simulink model "Systeem_Identificatie_Hardware_Code"  (R2018b)
settings: Solver=FixedStepDiscrete  StartTime=0.0  StopTime=1000  FixedStep=1/100000  RelTol=1e-3  EnableMultiTasking=on
libraries: mbedblockslib x3, dspswit3 x1, stm32f7lib x1
settings Model: Creator=Roberto  LastModifiedBy=Roberto
settings SolverCC: AutoInsertRateTranBlk=on
settings DataIOCC: SaveTime=off
settings OptimizationCC: DefaultParameterBehavior=Inlined  UseDivisionForNetSlopeComputation=on  UseFloatMulNetSlope=on  UseSpecifiedMinMax=on  InlineInvariantSignals=on  PassReuseOutputArgsAs=Individual arguments  ZeroExternalMemoryAtStartup=off  ZeroInternalMemoryAtStartup=off  NoFixptDivByZeroProtection=on  EfficientFloat2IntCast=on  LifeSpan=1  MaxStackSize=64  OptimizeBlockOrder=speed  DifferentSizesBufferReuse=on
settings DebuggingCC: ParameterTunabilityLossMsg=error
settings HardwareCC: ProdBitPerPointer=32  ProdBitPerSizeT=32  ProdBitPerPtrDiffT=32  ProdLargestAtomicInteger=Long  ProdLargestAtomicFloat=Double  ProdWordSize=32  ProdLongLongMode=on  ProdHWDeviceType=ARM Compatible->ARM Cortex
settings SFSimCC: MATLABDynamicMemAlloc=off
settings RTWCC: SystemTargetFile=ert.tlc  HardwareBoard=STM32F746G-Discovery  TemplateMakefile=ert_default_tmf  GenerateReport=on  Toolchain=GNU Tools for ARM Embedded Processors  BuildConfiguration=Faster Runs  IncludeHyperlinkInReport=on  LaunchReport=on  GenerateTraceInfo=on  GenerateTraceReport=on  GenerateTraceReportSl=on  GenerateTraceReportSf=on  GenerateTraceReportEml=on  GenerateCodeMetricsReport=on
settings CodeAppCC: ForceParamTrailComments=on  IgnoreCustomStorageClasses=off  OperatorAnnotations=on  SimulinkDataObjDesc=on  SFDataObjDesc=on  CustomSymbolStrGlobalVar=rt$N$M  CustomSymbolStrType=$N$M  CustomSymbolStrFcn=$N$M$F  CustomSymbolStrMacro=$N$M  InsertBlockDesc=on
settings ERTTargetCC: IncludeMdlTerminateFcn=off  CombineSignalStateStructs=on  SuppressErrorStatus=on  SupportNonFinite=off  SupportComplex=off  InlinedParameterPlacement=NonHierarchical  ERTFilePackagingFormat=CompactWithDataFile

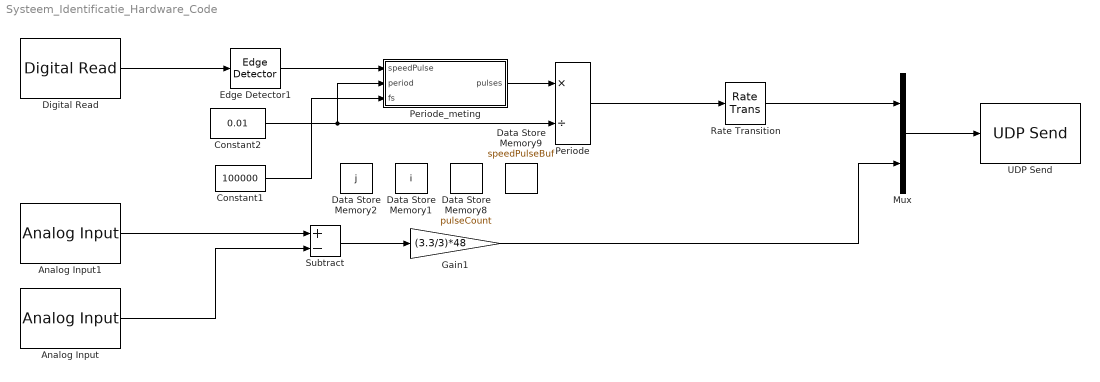
== system Systeem_Identificatie_Hardware_Code ==
  Analog Input : mbedblockslib/Analog Input  Pin=A1  ReadResultsOnly=off  ConversionTriggerSource=Software  ExternalTriggerType=uint32( 0 )  OutputDataType=double  EnableConversionCompleteNotify=off  EnableOuputStatus=off  SampleTime=1/50000
      settings: SourceProductName=Simulink Coder Support Package for BBC microbit Board  SourceProductBaseCode=MICROBIT
  Analog Input1 : mbedblockslib/Analog Input  Pin=A0  ReadResultsOnly=off  ConversionTriggerSource=Software  ExternalTriggerType=uint32( 0 )  OutputDataType=double  EnableConversionCompleteNotify=off  EnableOuputStatus=off  SampleTime=1/50000
      settings: SourceProductName=Simulink Coder Support Package for BBC microbit Board  SourceProductBaseCode=MICROBIT
  Constant1 : Constant  Value=100000
  Constant2 : Constant  Value=0.01
  Data Store Memory1 : DataStoreMemory  DataStoreName=i  ReadBeforeWriteMsg=warning  WriteAfterWriteMsg=warning  WriteAfterReadMsg=warning  InitialValue=1  ShowAdditionalParam=off  OutDataTypeStr=uint32
  Data Store Memory2 : DataStoreMemory  DataStoreName=j  ReadBeforeWriteMsg=warning  WriteAfterWriteMsg=warning  WriteAfterReadMsg=warning  InitialValue=2  ShowAdditionalParam=off  OutDataTypeStr=uint32
  Data Store Memory8 : DataStoreMemory  DataStoreName=pulseCount  ReadBeforeWriteMsg=warning  WriteAfterWriteMsg=warning  WriteAfterReadMsg=warning  ShowAdditionalParam=off  OutDataTypeStr=uint32
  Data Store Memory9 : DataStoreMemory  DataStoreName=speedPulseBuf  ReadBeforeWriteMsg=warning  WriteAfterWriteMsg=warning  WriteAfterReadMsg=warning  ShowAdditionalParam=off  OutDataTypeStr=uint8  Dimensions=1001
  Digital Read : mbedblockslib/Digital Read  Pin=2  Direction=input  SampleTime=1/100000
      settings: SourceProductName=Simulink Coder Support Package for BBC microbit Board  SourceProductBaseCode=MICROBIT
  Edge Detector1 : dspswit3/Edge Detector
      settings: SourceProductName=DSP System Toolbox  SourceProductBaseCode=DS
  Gain1 : Gain  Gain=(3.3/3)*48
  Mux : Mux  Inputs=2
  Periode : Product  Inputs=*/
  Periode_meting : MATLAB Function  TreatAsAtomicUnit=on
  Rate Transition : RateTransition  OutPortSampleTime=1/50000
  Subtract : Sum  Inputs=+-
  UDP Send : stm32f7lib/UDP Send  RemoteIPAddress_=255.255.255.255  RemoteIPPort_=25002  LocalIPPort_=-1  BlockingMode=on
      settings: SourceProductName=Embedded Coder Support Package for STMicroelectronics Discovery Boards  SourceProductBaseCode=STMICRODIS
  wires:
  Constant1/1 -> Periode_meting/3(fs)
  Constant2/1 -> Periode/2, Periode_meting/2(period)
  Periode_meting/1(pulses) -> Periode/1
  Edge Detector1/1 -> Periode_meting/1(speedPulse)
  Digital Read/1 -> Edge Detector1/1
  Periode/1 -> Rate Transition/1
  Mux/1 -> UDP Send/1
  Rate Transition/1 -> Mux/1
  Subtract/1 -> Gain1/1
  Analog Input/1 -> Subtract/2
  Analog Input1/1 -> Subtract/1
  Gain1/1 -> Mux/2

== matlab function Systeem_Identificatie_Hardware_Code/Periode_meting ==
  data: speedPulse input; pulses output; speedPulseBuf data_store_memory; pulseCount data_store_memory; period input; i data_store_memory; fs input; j data_store_memory
function pulses = fcn(speedPulse,period, fs)

global pulseCount;
global speedPulseBuf;
global i;
global j;

bufTime = period*fs + 1;

if i > bufTime
    i = uint32(1);
end

if j > bufTime
    j = uint32(1);
end

speedPulseBuf(i) = speedPulse;
pulseCount = pulseCount + uint32(speedPulse);
pulseCount = pulseCount - uint32(speedPulseBuf(j));

i = i + 1;
j = j + 1;

pulses = pulseCount;
